simulink model "testdemo"  (R2014b)
settings: Solver=ode45  StartTime=0.0  StopTime=10.0  RelTol=1e-3
settings Model: Creator=treasersmac  LastModifiedBy=treasersmac

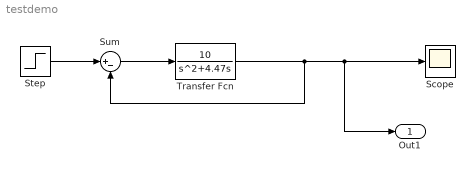
== system testdemo ==
  Scope : Scope
  Step : Step  SampleTime=0
  Sum : Sum  Inputs=|+-
  Transfer Fcn : TransferFcn  Numerator=[10]  Denominator=[1 4.47 0]
  Out1 : Outport
  wires:
  Transfer Fcn/1 -> Sum/2, Out1/1, Scope/1
  Step/1 -> Sum/1
  Sum/1 -> Transfer Fcn/1
